simulink library "EBCAN"  (R2017a)
settings: Solver=VariableStepAuto  StartTime=0.0  StopTime=10.0  RelTol=1e-3
settings Model: Creator=Di Russo  LastModifiedBy=Vraj M

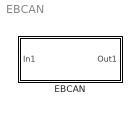
== system EBCAN ==
  EBCAN : Subsystem

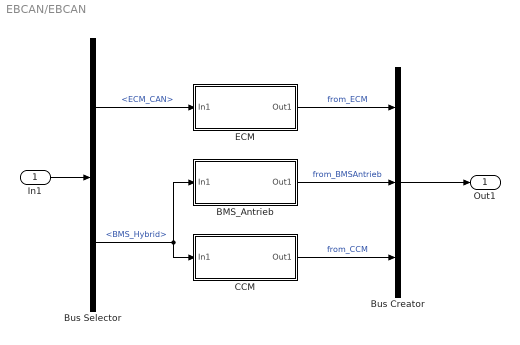
== system EBCAN/EBCAN ==
  In1 : Inport
  BMS_Antrieb : Subsystem
  Bus Creator : BusCreator  Inputs=3
  Bus Selector : BusSelector  OutputSignals=ECM_CAN,BMS_CAN.BMS_Hybrid
  CCM : Subsystem
  ECM : Subsystem
  Out1 : Outport
  wires:
  ECM/1(Out1) -> Bus Creator/1  "from_ECM"
  BMS_Antrieb/1(Out1) -> Bus Creator/2  "from_BMSAntrieb"
  Bus Creator/1 -> Out1/1
  CCM/1(Out1) -> Bus Creator/3  "from_CCM"
  In1/1 -> Bus Selector/1
  Bus Selector/1 -> ECM/1(In1)  "<ECM_CAN>"
  Bus Selector/2 -> CCM/1(In1), BMS_Antrieb/1(In1)  "<BMS_Hybrid>"

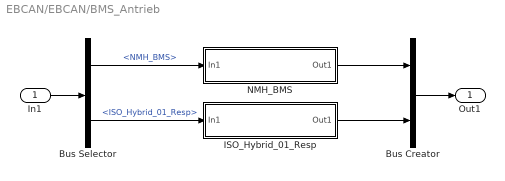
== system EBCAN/EBCAN/BMS_Antrieb ==
  In1 : Inport
  Bus Creator : BusCreator  Inputs=2
  Bus Selector : BusSelector  OutputSignals=NMH_BMS,ISO_Hybrid_01_Resp
  ISO_Hybrid_01_Resp : Subsystem
  NMH_BMS : Subsystem
  Out1 : Outport
  wires:
  In1/1 -> Bus Selector/1
  Bus Selector/1 -> NMH_BMS/1(In1)  "<NMH_BMS>"
  NMH_BMS/1(Out1) -> Bus Creator/1
  ISO_Hybrid_01_Resp/1(Out1) -> Bus Creator/2
  Bus Creator/1 -> Out1/1
  Bus Selector/2 -> ISO_Hybrid_01_Resp/1(In1)  "<ISO_Hybrid_01_Resp>"

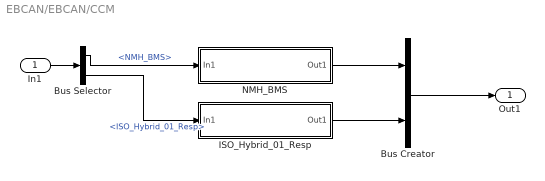
== system EBCAN/EBCAN/CCM ==
  In1 : Inport
  Bus Creator : BusCreator  Inputs=2
  Bus Selector : BusSelector  OutputSignals=NMH_BMS,ISO_Hybrid_01_Resp
  ISO_Hybrid_01_Resp : Subsystem
  NMH_BMS : Subsystem
  Out1 : Outport
  wires:
  Bus Selector/2 -> ISO_Hybrid_01_Resp/1(In1)  "<ISO_Hybrid_01_Resp>"
  Bus Creator/1 -> Out1/1
  ISO_Hybrid_01_Resp/1(Out1) -> Bus Creator/2
  NMH_BMS/1(Out1) -> Bus Creator/1
  Bus Selector/1 -> NMH_BMS/1(In1)  "<NMH_BMS>"
  In1/1 -> Bus Selector/1

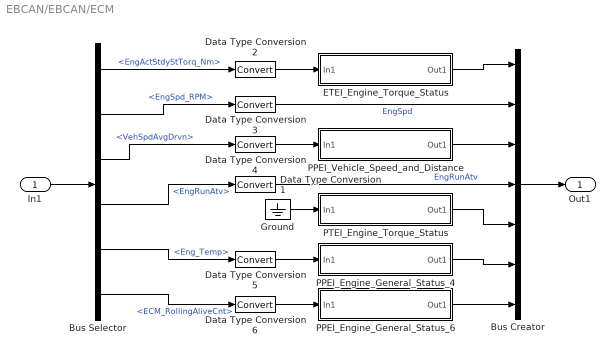
== system EBCAN/EBCAN/ECM ==
  In1 : Inport
  Bus Creator : BusCreator  Inputs=7
  Bus Selector : BusSelector  OutputSignals=Sensors_to_ECM.EngActStdyStTorq_Nm,Sensors_to_ECM.EngSpd_RPM,ECM_to_Actuators.VehSpdAvgDrvn,ECM_to_Actuators.EngRunAtv,ECM_to_Actuators.Eng_Temp,ECM_to_Actuators.ECM_RollingAliveCnt
  Data Type Conversion{1..6} (6 alike) : DataTypeConversion
  ETEI_Engine_Torque_Status : Subsystem
  Ground : Ground
  PPEI_Engine_General_Status_4 : Subsystem
  PPEI_Engine_General_Status_6 : Subsystem
  PPEI_Vehicle_Speed_and_Distance : Subsystem
  PTEI_Engine_Torque_Status : Subsystem
  Out1 : Outport
  wires:
  Bus Selector/6 -> Data Type Conversion6/1  "<ECM_RollingAliveCnt>"
  Bus Selector/5 -> Data Type Conversion5/1  "<Eng_Temp>"
  Bus Selector/3 -> Data Type Conversion4/1  "<VehSpdAvgDrvn>"
  Bus Selector/1 -> Data Type Conversion2/1  "<EngActStdyStTorq_Nm>"
  In1/1 -> Bus Selector/1
  Data Type Conversion2/1 -> ETEI_Engine_Torque_Status/1(In1)
  Bus Selector/2 -> Data Type Conversion3/1  "<EngSpd_RPM>"
  Data Type Conversion4/1 -> PPEI_Vehicle_Speed_and_Distance/1(In1)
  ETEI_Engine_Torque_Status/1(Out1) -> Bus Creator/1
  PPEI_Vehicle_Speed_and_Distance/1(Out1) -> Bus Creator/3
  Bus Creator/1 -> Out1/1
  Bus Selector/4 -> Data Type Conversion1/1  "<EngRunAtv>"
  Ground/1 -> PTEI_Engine_Torque_Status/1(In1)
  PTEI_Engine_Torque_Status/1(Out1) -> Bus Creator/5
  Data Type Conversion5/1 -> PPEI_Engine_General_Status_4/1(In1)
  PPEI_Engine_General_Status_4/1(Out1) -> Bus Creator/6
  Data Type Conversion6/1 -> PPEI_Engine_General_Status_6/1(In1)
  PPEI_Engine_General_Status_6/1(Out1) -> Bus Creator/7
  Data Type Conversion3/1 -> Bus Creator/2  "EngSpd"
  Data Type Conversion1/1 -> Bus Creator/4  "EngRunAtv"

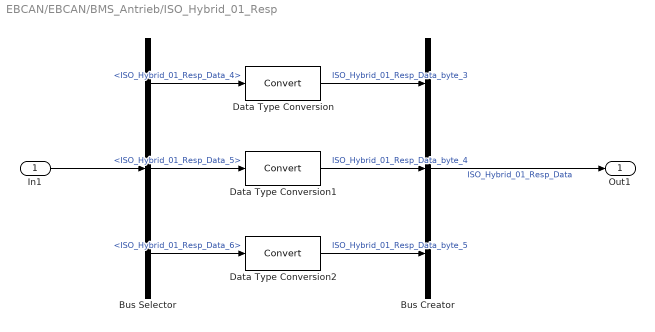
== system EBCAN/EBCAN/BMS_Antrieb/ISO_Hybrid_01_Resp ==
  In1 : Inport
  Bus Creator : BusCreator  Inputs=3
  Bus Selector : BusSelector  OutputSignals=ISO_Hybrid_01_Resp_Data_4,ISO_Hybrid_01_Resp_Data_5,ISO_Hybrid_01_Resp_Data_6
  Data Type Conversion : DataTypeConversion
  Data Type Conversion1 : DataTypeConversion
  Data Type Conversion2 : DataTypeConversion
  Out1 : Outport
  wires:
  Data Type Conversion2/1 -> Bus Creator/3  "ISO_Hybrid_01_Resp_Data_byte_5"
  Data Type Conversion1/1 -> Bus Creator/2  "ISO_Hybrid_01_Resp_Data_byte_4"
  Data Type Conversion/1 -> Bus Creator/1  "ISO_Hybrid_01_Resp_Data_byte_3"
  Bus Creator/1 -> Out1/1  "ISO_Hybrid_01_Resp_Data"
  Bus Selector/3 -> Data Type Conversion2/1  "<ISO_Hybrid_01_Resp_Data_6>"
  Bus Selector/2 -> Data Type Conversion1/1  "<ISO_Hybrid_01_Resp_Data_5>"
  Bus Selector/1 -> Data Type Conversion/1  "<ISO_Hybrid_01_Resp_Data_4>"
  In1/1 -> Bus Selector/1

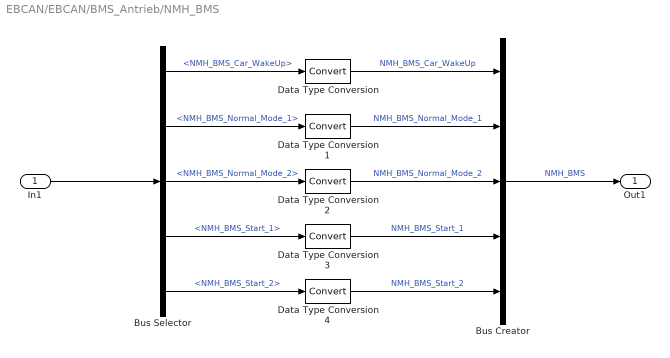
== system EBCAN/EBCAN/BMS_Antrieb/NMH_BMS ==
  In1 : Inport
  Bus Creator : BusCreator  Inputs=5
  Bus Selector : BusSelector  OutputSignals=NMH_BMS_Car_WakeUp,NMH_BMS_Normal_Mode_1,NMH_BMS_Normal_Mode_2,NMH_BMS_Start_1,NMH_BMS_Start_2
  Data Type Conversion{,1..4} (5 alike) : DataTypeConversion
  Out1 : Outport
  wires:
  Data Type Conversion4/1 -> Bus Creator/5  "NMH_BMS_Start_2"
  Data Type Conversion3/1 -> Bus Creator/4  "NMH_BMS_Start_1"
  Data Type Conversion2/1 -> Bus Creator/3  "NMH_BMS_Normal_Mode_2"
  Data Type Conversion1/1 -> Bus Creator/2  "NMH_BMS_Normal_Mode_1"
  Data Type Conversion/1 -> Bus Creator/1  "NMH_BMS_Car_WakeUp"
  Bus Selector/1 -> Data Type Conversion/1  "<NMH_BMS_Car_WakeUp>"
  Bus Selector/2 -> Data Type Conversion1/1  "<NMH_BMS_Normal_Mode_1>"
  Bus Selector/3 -> Data Type Conversion2/1  "<NMH_BMS_Normal_Mode_2>"
  Bus Selector/4 -> Data Type Conversion3/1  "<NMH_BMS_Start_1>"
  Bus Selector/5 -> Data Type Conversion4/1  "<NMH_BMS_Start_2>"
  Bus Creator/1 -> Out1/1  "NMH_BMS"
  In1/1 -> Bus Selector/1

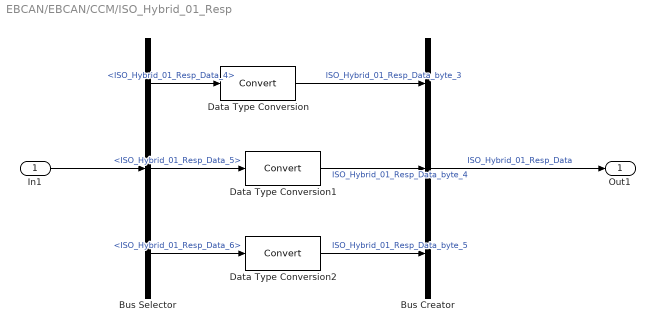
== system EBCAN/EBCAN/CCM/ISO_Hybrid_01_Resp ==
  In1 : Inport
  Bus Creator : BusCreator  Inputs=3
  Bus Selector : BusSelector  OutputSignals=ISO_Hybrid_01_Resp_Data_4,ISO_Hybrid_01_Resp_Data_5,ISO_Hybrid_01_Resp_Data_6
  Data Type Conversion : DataTypeConversion
  Data Type Conversion1 : DataTypeConversion
  Data Type Conversion2 : DataTypeConversion
  Out1 : Outport
  wires:
  In1/1 -> Bus Selector/1
  Bus Selector/1 -> Data Type Conversion/1  "<ISO_Hybrid_01_Resp_Data_4>"
  Bus Selector/2 -> Data Type Conversion1/1  "<ISO_Hybrid_01_Resp_Data_5>"
  Bus Selector/3 -> Data Type Conversion2/1  "<ISO_Hybrid_01_Resp_Data_6>"
  Bus Creator/1 -> Out1/1  "ISO_Hybrid_01_Resp_Data"
  Data Type Conversion/1 -> Bus Creator/1  "ISO_Hybrid_01_Resp_Data_byte_3"
  Data Type Conversion1/1 -> Bus Creator/2  "ISO_Hybrid_01_Resp_Data_byte_4"
  Data Type Conversion2/1 -> Bus Creator/3  "ISO_Hybrid_01_Resp_Data_byte_5"

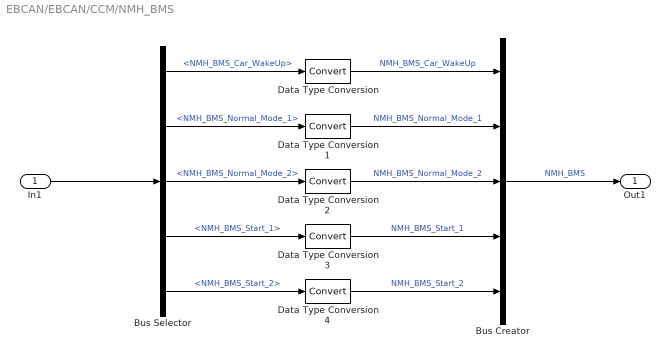
== system EBCAN/EBCAN/CCM/NMH_BMS ==
  In1 : Inport
  Bus Creator : BusCreator  Inputs=5
  Bus Selector : BusSelector  OutputSignals=NMH_BMS_Car_WakeUp,NMH_BMS_Normal_Mode_1,NMH_BMS_Normal_Mode_2,NMH_BMS_Start_1,NMH_BMS_Start_2
  Data Type Conversion{,1..4} (5 alike) : DataTypeConversion
  Out1 : Outport
  wires:
  In1/1 -> Bus Selector/1
  Bus Creator/1 -> Out1/1  "NMH_BMS"
  Bus Selector/5 -> Data Type Conversion4/1  "<NMH_BMS_Start_2>"
  Bus Selector/4 -> Data Type Conversion3/1  "<NMH_BMS_Start_1>"
  Bus Selector/3 -> Data Type Conversion2/1  "<NMH_BMS_Normal_Mode_2>"
  Bus Selector/2 -> Data Type Conversion1/1  "<NMH_BMS_Normal_Mode_1>"
  Bus Selector/1 -> Data Type Conversion/1  "<NMH_BMS_Car_WakeUp>"
  Data Type Conversion/1 -> Bus Creator/1  "NMH_BMS_Car_WakeUp"
  Data Type Conversion1/1 -> Bus Creator/2  "NMH_BMS_Normal_Mode_1"
  Data Type Conversion2/1 -> Bus Creator/3  "NMH_BMS_Normal_Mode_2"
  Data Type Conversion3/1 -> Bus Creator/4  "NMH_BMS_Start_1"
  Data Type Conversion4/1 -> Bus Creator/5  "NMH_BMS_Start_2"

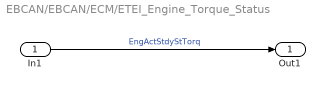
== system EBCAN/EBCAN/ECM/ETEI_Engine_Torque_Status ==
  In1 : Inport
  Out1 : Outport
  wires:
  In1/1 -> Out1/1  "EngActStdyStTorq"

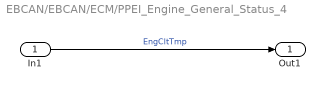
== system EBCAN/EBCAN/ECM/PPEI_Engine_General_Status_4 ==
  In1 : Inport
  Out1 : Outport
  wires:
  In1/1 -> Out1/1  "EngCltTmp"

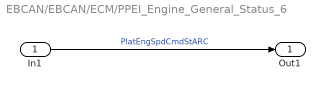
== system EBCAN/EBCAN/ECM/PPEI_Engine_General_Status_6 ==
  In1 : Inport
  Out1 : Outport
  wires:
  In1/1 -> Out1/1  "PlatEngSpdCmdStARC"

== system EBCAN/EBCAN/ECM/PPEI_Vehicle_Speed_and_Distance ==
  In1 : Inport
  Out1 : Outport
  wires:
  In1/1 -> Out1/1  "VehSpdAvgDrvn"

== system EBCAN/EBCAN/ECM/PTEI_Engine_Torque_Status ==
  In1 : Inport
  Out1 : Outport
  wires:
  In1/1 -> Out1/1  "CrksftNTrnsRegCmdTq"
